simulink model "practice6_1"  (Simulink 7.9)
settings: Solver=ode45  StartTime=0.0  StopTime=200  RelTol=1e-3
settings Model: Creator=sony  LastModifiedBy=sony

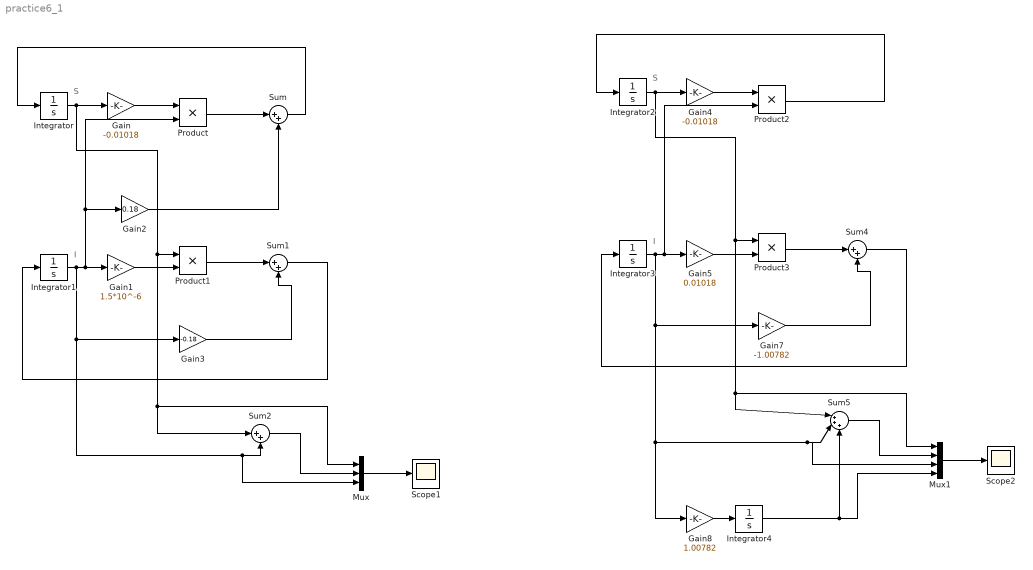
== system practice6_1 ==
  note: S
  note: I
  note: S
  note: I
  Gain : Gain  Gain=-0.01018
  Gain1 : Gain  Gain=1.5*10^-6
  Gain2 : Gain  Gain=0.18
  Gain3 : Gain  Gain=-0.18
  Gain4 : Gain  Gain=-0.01018
  Gain5 : Gain  Gain=0.01018
  Gain7 : Gain  Gain=-1.00782
  Gain8 : Gain  Gain=1.00782
  Integrator : Integrator  InitialCondition=99
  Integrator1 : Integrator  InitialCondition=1
  Integrator2 : Integrator  InitialCondition=99
  Integrator3 : Integrator  InitialCondition=1
  Integrator4 : Integrator
  Mux : Mux  Inputs=3
  Mux1 : Mux
  Product{,1..3} (4 alike) : Product  RndMeth=Zero
  Scope1 : Scope
      settings: TimeRange=10
  Scope2 : Scope
      settings: TimeRange=10
  Sum{,1..2,4} (4 alike) : Sum  Inputs=|++
  Sum5 : Sum  Inputs=|+++
  wires:
  Integrator1/1 -> Gain1/1, Product/2, Gain2/1, Gain3/1, Sum2/2, Mux/3
  Integrator/1 -> Gain/1, Product1/1, Sum2/1, Mux/1
  Gain/1 -> Product/1
  Product/1 -> Sum/1
  Gain2/1 -> Sum/2
  Sum/1 -> Integrator/1
  Gain1/1 -> Product1/2
  Product1/1 -> Sum1/1
  Gain3/1 -> Sum1/2
  Sum1/1 -> Integrator1/1
  Sum2/1 -> Mux/2
  Mux/1 -> Scope1/1
  Integrator3/1 -> Gain5/1, Product2/2, Gain7/1, Gain8/1, Mux1/3, Sum5/2
  Integrator2/1 -> Gain4/1, Product3/1, Sum5/1, Mux1/1
  Gain4/1 -> Product2/1
  Product2/1 -> Integrator2/1
  Gain5/1 -> Product3/2
  Product3/1 -> Sum4/1
  Gain7/1 -> Sum4/2
  Sum4/1 -> Integrator3/1
  Sum5/1 -> Mux1/2
  Mux1/1 -> Scope2/1
  Gain8/1 -> Integrator4/1
  Integrator4/1 -> Sum5/3, Mux1/4
